simulink model "watertank_simulation"  (R2025b)
settings: Solver=FixedStepAuto  StartTime=0.0  StopTime=600  FixedStep=.005  MaxStep=1e-4  RelTol=1e-3
libraries: simulink x1, slpidlib x1
settings Model: Creator=Simon  LastModifiedBy=Felix
settings HardwareCC: ProdHWDeviceType=AMD->x86-64 (Windows64)

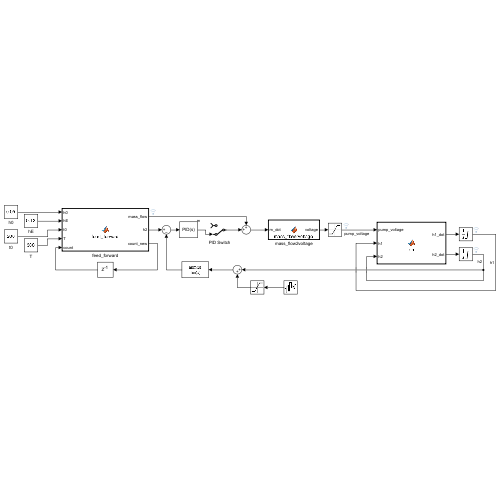
[thumbnail: Simulink's stored preview of the top-level diagram]
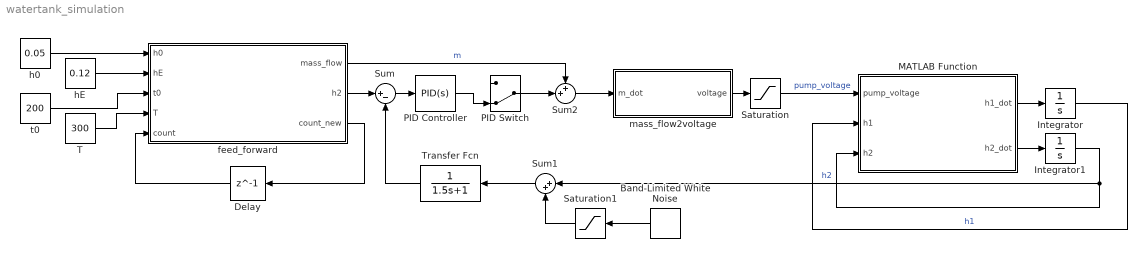
== system watertank_simulation ==
  Band-Limited White Noise : simulink/Sources/Band-Limited White Noise  Cov=[0.01]  Ts=0.1  seed=[23341]
  Delay : Delay  DelayLength=1
  Integrator : Integrator  LimitOutput=on  UpperSaturationLimit=.3  LowerSaturationLimit=0
  Integrator1 : Integrator  LimitOutput=on  UpperSaturationLimit=.3  LowerSaturationLimit=0
  MATLAB Function : MATLAB Function  TreatAsAtomicUnit=on
  PID Controller : slpidlib/PID Controller  Controller=PID  Form=Parallel  TimeDomain=Continuous-time  UseExternalTs=off  SampleTime=-1  IntegratorMethod=Forward Euler  FilterMethod=Forward Euler  ControllerParametersSource=internal  P=.9417  I=.04159  UseKiTs=off  D=5.331  UseExternalDerivativeSource=off  N=100  UseFilter=on  TunerSelectOption=Transfer Function Based (PID Tuner App)  InitialConditionSource=internal  InitialConditionForIntegrator=0  InitialConditionForFilter=0  DifferentiatorICPrevScaledInput=0  ExternalReset=none  TrackingMode=off  Kt=1  LimitOutput=off  SatLimitsSource=internal  UpperSaturationLimit=inf  LowerSaturationLimit=-inf  LinearizeAsGain=on  AntiWindupMode=none  Kb=1  LimitIntegrator=off  UpperIntegratorSaturationLimit=inf  LowerIntegratorSaturationLimit=-inf  POutMin=[]  POutMax=[]  IOutMin=[]  IOutMax=[]  DOutMin=[]  DOutMax=[]  NOutMin=[]  NOutMax=[]  SumOutMin=[]  SumOutMax=[]  SaturationOutMin=[]  SaturationOutMax=[]  PParamMin=[]  PParamMax=[]  IParamMin=[]  IParamMax=[]  DParamMin=[]  DParamMax=[]  NParamMin=[]  NParamMax=[]  KbParamMin=[]  KbParamMax=[]  KtParamMin=[]  KtParamMax=[]  KbOutMin=[]  KbOutMax=[]  KtOutMin=[]  KtOutMax=[]  IntegratorOutMin=[]  IntegratorOutMax=[]  FilterOutMin=[]  FilterOutMax=[]  SumI1OutMin=[]  SumI1OutMax=[]  SumI2OutMin=[]  SumI2OutMax=[]  SumI3OutMin=[]  SumI3OutMax=[]  SumI4OutMin=[]  SumI4OutMax=[]  SumDOutMin=[]  SumDOutMax=[]  DifferentiatorOutMin=[]  DifferentiatorOutMax=[]  FilterDiffOutCoefMin=[]  FilterDiffOutCoefMax=[]  ReciprocalOutMin=[]  ReciprocalOutMax=[]  SumDenOutMin=[]  SumDenOutMax=[]  SumNumOutMin=[]  SumNumOutMax=[]  DivideOutMin=[]  DivideOutMax=[]  UdiffTsProdOutMin=[]  UdiffTsProdOutMax=[]  NTsProdOutMin=[]  NTsProdOutMax=[]  UintegralTsProdOutMin=[]  UintegralTsProdOutMax=[]  UngainTsProdOutMin=[]  UngainTsProdOutMax=[]  ClampingZeroOutDataTypeStr=Inherit: Inherit via back propagation  ClampingZeroOutMin=[]  ClampingZeroOutMax=[]  FilterDenConstantOutDataTypeStr=Inherit: Inherit via back propagation  FilterDenConstantOutMin=[]  FilterDenConstantOutMax=[]  PCopyOutDataTypeStr=Inherit: Inherit via back propagation  PCopyOutMin=[]  PCopyOutMax=[]  NCopyOutDataTypeStr=Inherit: Inherit via back propagation  NCopyOutMin=[]  NCopyOutMax=[]  IntegratorContinuousStateAttributes=''  IntegratorStateMustResolveToSignalObject=off  IntegratorRTWStateStorageClass=Auto  FilterContinuousStateAttributes=''  FilterStateMustResolveToSignalObject=off  FilterRTWStateStorageClass=Auto  ParallelPVariant=InternalParameters  IdealPVariant=Disabled  IVariant=InternalParameters  DVariant=InternalParameters  IntegratorVariant=Continuous  SatVariant=Disabled  AWVariant=Passthrough  PCopyVariant=Disabled  TRVariant=Disabled  FdbkBlocksVariant=Forward  IdealPFdbkVariant=Disabled  SatFdbkVariant=Disabled  DerivativeFilterVariant=ContFilter  NVariant=InternalParameters  NCopyVariant=Disabled  FilterICVariant=InternalICsFilter  IntegratorICVariant=InternalICs  ExternalResetVariant=Disabled  TRSumVariant=Passthrough  SumFdbkVariant=Disabled  SumVariant=Sum_PID  TsampFilterVariant=InternalTs  TsampNgainVariant=Passthrough  TsampIntegralVariant=Disabled_SignalSpec  ExternalSaturationOutDataTypeStr=Inherit: Same as second input  DerivativeSourceVariant=ErrorSignal  PreIntVariant=InternalPreInt
  PID Switch : ManualSwitch  CurrentSetting=0
  Saturation : Saturate  UpperLimit=5  LowerLimit=0
  Saturation1 : Saturate  UpperLimit=0.01  LowerLimit=-0.01
  Sum : Sum  Inputs=|+-
  Sum1 : Sum  Inputs=|++
  Sum2 : Sum  Inputs=++|
  T : Constant  Value=300
  Transfer Fcn : TransferFcn  Denominator=[1.5 1]
  feed_forward : MATLAB Function  TreatAsAtomicUnit=on
  h0 : Constant  Value=0.05
  hE : Constant  Value=0.12
  mass_flow2voltage : MATLAB Function  TreatAsAtomicUnit=on
  t0 : Constant  Value=200
  wires:
  MATLAB Function/1(h1_dot) -> Integrator/1
  MATLAB Function/2(h2_dot) -> Integrator1/1
  Integrator/1 -> MATLAB Function/2(h1)  "h1"
  Integrator1/1 -> Sum1/1, MATLAB Function/3(h2)  "h2"
  Sum/1 -> PID Controller/1
  mass_flow2voltage/1(voltage) -> Saturation/1
  Band-Limited White Noise/1 -> Saturation1/1
  Saturation1/1 -> Sum1/2
  Transfer Fcn/1 -> Sum/2
  t0/1 -> feed_forward/3(t0)
  T/1 -> feed_forward/4(T)
  h0/1 -> feed_forward/1(h0)
  hE/1 -> feed_forward/2(hE)
  feed_forward/3(count_new) -> Delay/1
  Delay/1 -> feed_forward/5(count)
  feed_forward/2(h2) -> Sum/1
  Sum2/1 -> mass_flow2voltage/1(m_dot)
  feed_forward/1(mass_flow) -> Sum2/1  "m"
  PID Controller/1 -> PID Switch/2
  PID Switch/1 -> Sum2/2
  Sum1/1 -> Transfer Fcn/1
  Saturation/1 -> MATLAB Function/1(pump_voltage)  "pump_voltage"

== matlab function watertank_simulation/mass_flow2voltage ==
  data: m_dot input; voltage output
function voltage = mass_flow2voltage(m_dot)
K_pump = 0.0167;
u0_pump = 0.25;
voltage = (m_dot/K_pump) + u0_pump;

== matlab function watertank_simulation/MATLAB Function ==
  data: pump_voltage input; h1_dot output; h2_dot output; h1 input; h2 input
function [h1_dot,h2_dot]= fcn(pump_voltage, h1, h2)
K_pump = 0.0167;
u0_pump = 0.25;
mass_flow1 = K_pump * (pump_voltage - u0_pump);

a1 = 0.0574;
a2 = 0.0524;

rho = 1000;
A_t = 0.005;

h1 = max(0, h1);
h2 = max(0, h2);

h1_dot = (-a1 * sqrt(h1)) + (1 / (rho * A_t)) * mass_flow1;

h2_dot = (a1 * sqrt(h1) - a2 * sqrt(h2));

== matlab function watertank_simulation/feed_forward ==
  data: mass_flow output; h2 output; h0 input; hE input; t0 input; T input; count input; count_new output
function [mass_flow, h2, count_new] = feed_forward(h0,hE,t0,T,count)
count_new = count+1;
dT = 0.005;
t = count_new*dT-t0;
h2 = 0;
h2_dot = 0;
h2_ddot = 0;

a1 = 0.0574;
a2 = 0.0524;
rho = 1000;
At = 50e-4;
if t<0
    h2 = h0;
elseif t>T
    h2 = hE;
else
    % Trajectory
    tau = t / T;
    dh = hE - h0;

    h2 = h0 + dh * (10 * tau^3 - 15 * tau^4 + 6 * tau^5);
    h2_dot = dh * (30 * tau^2 - 60 * tau^3 + 30 * tau^4) / T;
    h2_ddot = dh * (60 * tau - 180 * tau^2 + 120 * tau^3) / (T^2);
end
h2_safe = max(h2, 1e-12);
h1 = ((h2_dot + a2 * sqrt(h2)) / a1)^2; 
h1_dot = (2 * sqrt(h1) / a1) * (h2_ddot + (a2 * h2_dot) / (2 * sqrt(h2_safe)));
mass_flow = max(0, (h1_dot + a1 * sqrt(h1)) * rho * At); 
end
